simulink model "Sim_q5"  (Simulink 8.1)
settings: Solver=ode45  StartTime=0.0  StopTime=Tend  MaxStep=dt  RelTol=1e-3
InitFcn:
  | A=3;
  | a=0.75;
  | b=0.1
  | T=0.2;
  | Tend=50;
  | dt=1/100;
StopFcn:
  | close all;
  | t=Dados.time;
  | ref=Dados.signals.values(:,1);
  | es=Dados.signals.values(:,2);
  | y=Dados.signals.values(:,3);
  | ys=Dados.signals.values(:,4);
  | plot(t,ref,'k-',t,y,'r-'); hold on;
  | stairs(t,ys,'b-');
  | xlabel('t (s)');
  | legend('Ref(t)','Y(t)','Ys(t)');
  | title(['T = ', num2str(T), ' s']);
  | grid;
settings Model: Creator=cairo  LastModifiedBy=cairo

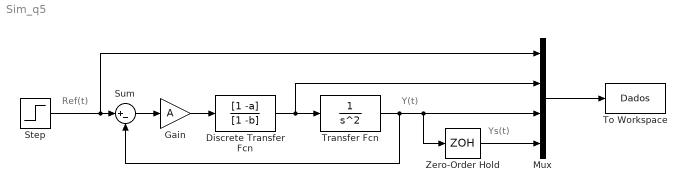
== system Sim_q5 ==
  note: Ref(t)
  note: Y(t)
  note: Ys(t)
  Discrete Transfer Fcn : DiscreteTransferFcn  Numerator=[1 -a]  Denominator=[1 -b]  SampleTime=T
  Gain : Gain  Gain=A
  Mux : Mux
  Step : Step  Time=0  SampleTime=0
  Sum : Sum  Inputs=|+-
  To Workspace : ToWorkspace  VariableName=Dados  SampleTime=-1  SaveFormat=Structure With Time
  Transfer Fcn : TransferFcn  Denominator=[1 0 0]
  Zero-Order Hold : ZeroOrderHold  SampleTime=T
  wires:
  Step/1 -> Sum/1, Mux/1
  Sum/1 -> Gain/1
  Discrete Transfer Fcn/1 -> Transfer Fcn/1, Mux/2
  Transfer Fcn/1 -> Sum/2, Mux/3, Zero-Order Hold/1
  Mux/1 -> To Workspace/1
  Zero-Order Hold/1 -> Mux/4
  Gain/1 -> Discrete Transfer Fcn/1
